simulink model "LF_AC29bus_HVDCdemo_V2_1"  (R2019b)
settings: Solver=FixedStepDiscrete  StartTime=0.0  StopTime=fix(6/Ts)*Ts  FixedStep=Ts  RelTol=1e-3
InitFcn:
  | Ts_avg=150e-6;
  | Ts=50e-6;
  | 
  | %Tc_stab = 1/60/5;
  | %Tc_stab = 2/60;
  | Tc_stab = Ts;
  | 
  | 
  | Ts_avg=150e-6;
  | 
  | Ts=50e-6;
  | 
  | % Rectifier AC side :
  | VLL_nom_R = 735e3; % V
  | Fnom_R = 60;           % Hz
  | 
  | % Inverter AC side :
  | VLL_nom_I = 735e3; % V
  | Fnom_I = 60;           % Hz
  | 
  | % DC :
  | Vdc_nom = 500e3;   % V
  | Idc_nom  = 2000;     % A
undefined symbols (not defined in the file): D1, D11, Delta, test_alpha
libraries: powerlib x223, powerlib_meascontrol x57, simulink x22, sps_avr x7
(part 7 of 10)

== system LF_AC29bus_HVDCdemo_V2_1/North-West Network/Regulators2/Turbine  & Excitation Regulators Mac2 ==
  Pref : Inport
  Vref : Inport  Port=2
  Vm : Inport  Port=3
  w : Inport  Port=4
  Pe : Inport  Port=5
  Add : Sum  Inputs=+-
  Complex to Real-Imag : ComplexToRealImag
  Excitation System : sps_avr/Excitation System  tr=20e-3  reg=[ 300, 0.001 ]  exc=[ 1, 0 ]  tgr=[ 0, 0 ]  damp=[ 0.001, 0.1 ]  sat=[ 0, 0 ]  lim=[ -11.5, 11.5, 0 ]  v0=[1 1.33]
      settings: SourceProductName=Simscape Electrical  SourceProductBaseCode=PS
  Hydraulic Turbine and Governor : powerlib/Machines/Hydraulic Turbine and Governor  sm="[ 10/3  0.07 ]"  gate="[  0.01  0.97518  -0.1  0.1 ]"  reg="[  0.05 1.163  0.105  0  0.01  ]"  hyd="[  0  2.67  ]"  dref=0  po=0.82009
      settings: SourceProductName=Simscape Electrical  SourceProductBaseCode=PS
  Stabilisateur : Subsystem
  Terminator : Terminator
  wref : Constant
  wref1 : Constant
  Pm : Outport
  Vf : Outport  Port=2
  wires:
  Stabilisateur/1(Stab) -> Excitation System/4
  Add/1 -> Stabilisateur/3(dw), Hydraulic Turbine and Governor/5
  wref1/1 -> Add/2
  Complex to Real-Imag/1 -> Excitation System/2
  Complex to Real-Imag/2 -> Excitation System/3
  Vm/1 -> Complex to Real-Imag/1
  w/1 -> Add/1, Hydraulic Turbine and Governor/3
  wref/1 -> Hydraulic Turbine and Governor/1
  Vref/1 -> Excitation System/1
  Pref/1 -> Hydraulic Turbine and Governor/2
  Pe/1 -> Stabilisateur/2(Pe), Hydraulic Turbine and Governor/4
  Excitation System/1 -> Vf/1
  Hydraulic Turbine and Governor/1 -> Stabilisateur/1(Pm), Pm/1
  Hydraulic Turbine and Governor/2 -> Terminator/1

== system LF_AC29bus_HVDCdemo_V2_1/North-West Network/Regulators3/Turbine  & Excitation Regulators Mac2 ==
  Pref : Inport
  Vref : Inport  Port=2
  Vm : Inport  Port=3
  w : Inport  Port=4
  Pe : Inport  Port=5
  Add : Sum  Inputs=+-
  Complex to Real-Imag : ComplexToRealImag
  Excitation System : sps_avr/Excitation System  tr=20e-3  reg=[ 300, 0.001 ]  exc=[ 1, 0 ]  tgr=[ 0, 0 ]  damp=[ 0.001, 0.1 ]  sat=[ 0, 0 ]  lim=[ -11.5, 11.5, 0 ]  v0=[1 1.3999]
      settings: SourceProductName=Simscape Electrical  SourceProductBaseCode=PS
  Hydraulic Turbine and Governor : powerlib/Machines/Hydraulic Turbine and Governor  sm="[ 10/3  0.07 ]"  gate="[  0.01  0.97518  -0.1  0.1 ]"  reg="[  0.05 1.163  0.105  0  0.01  ]"  hyd="[  0  2.67  ]"  dref=0  po=0.90231
      settings: SourceProductName=Simscape Electrical  SourceProductBaseCode=PS
  Stabilisateur : Subsystem
  Terminator : Terminator
  wref : Constant
  wref1 : Constant
  Pm : Outport
  Vf : Outport  Port=2
  wires:
  Hydraulic Turbine and Governor/2 -> Terminator/1
  Hydraulic Turbine and Governor/1 -> Pm/1, Stabilisateur/1(Pm)
  Excitation System/1 -> Vf/1
  Pe/1 -> Hydraulic Turbine and Governor/4, Stabilisateur/2(Pe)
  Pref/1 -> Hydraulic Turbine and Governor/2
  Vref/1 -> Excitation System/1
  wref/1 -> Hydraulic Turbine and Governor/1
  w/1 -> Hydraulic Turbine and Governor/3, Add/1
  Vm/1 -> Complex to Real-Imag/1
  Complex to Real-Imag/2 -> Excitation System/3
  Complex to Real-Imag/1 -> Excitation System/2
  wref1/1 -> Add/2
  Add/1 -> Hydraulic Turbine and Governor/5, Stabilisateur/3(dw)
  Stabilisateur/1(Stab) -> Excitation System/4

== system LF_AC29bus_HVDCdemo_V2_1/North-West Network/Regulators4/Turbine  & Excitation Regulators Mac2 ==
  Pref : Inport
  Vref : Inport  Port=2
  Vm : Inport  Port=3
  w : Inport  Port=4
  Pe : Inport  Port=5
  Add : Sum  Inputs=+-
  Complex to Real-Imag : ComplexToRealImag
  Excitation System : sps_avr/Excitation System  tr=20e-3  reg=[ 300, 0.001 ]  exc=[ 1, 0 ]  tgr=[ 0, 0 ]  damp=[ 0.001, 0.1 ]  sat=[ 0, 0 ]  lim=[ -11.5, 11.5, 0 ]  v0=[1 1.3172]
      settings: SourceProductName=Simscape Electrical  SourceProductBaseCode=PS
  Hydraulic Turbine and Governor : powerlib/Machines/Hydraulic Turbine and Governor  sm="[ 10/3  0.07 ]"  gate="[  0.01  0.97518  -0.1  0.1 ]"  reg="[  0.05 1.163  0.105  0  0.01  ]"  hyd="[  0  2.67  ]"  dref=0  po=0.92839
      settings: SourceProductName=Simscape Electrical  SourceProductBaseCode=PS
  Stabilisateur : Subsystem
  Terminator : Terminator
  wref : Constant
  wref1 : Constant
  Pm : Outport
  Vf : Outport  Port=2
  wires:
  Stabilisateur/1(Stab) -> Excitation System/4
  Add/1 -> Stabilisateur/3(dw), Hydraulic Turbine and Governor/5
  wref1/1 -> Add/2
  Complex to Real-Imag/1 -> Excitation System/2
  Complex to Real-Imag/2 -> Excitation System/3
  Vm/1 -> Complex to Real-Imag/1
  w/1 -> Add/1, Hydraulic Turbine and Governor/3
  wref/1 -> Hydraulic Turbine and Governor/1
  Vref/1 -> Excitation System/1
  Pref/1 -> Hydraulic Turbine and Governor/2
  Pe/1 -> Stabilisateur/2(Pe), Hydraulic Turbine and Governor/4
  Excitation System/1 -> Vf/1
  Hydraulic Turbine and Governor/1 -> Stabilisateur/1(Pm), Pm/1
  Hydraulic Turbine and Governor/2 -> Terminator/1

== system LF_AC29bus_HVDCdemo_V2_1/North_East Network/Regulateurs6/Turbine  & Excitation Regulators Mac2 ==
  Pref : Inport
  Vref : Inport  Port=2
  Vm : Inport  Port=3
  w : Inport  Port=4
  Pe : Inport  Port=5
  Add : Sum  Inputs=+-
  Complex to Real-Imag : ComplexToRealImag
  Excitation System : sps_avr/Excitation System  tr=20e-3  reg=[ 300, 0.001 ]  exc=[ 1, 0 ]  tgr=[ 0, 0 ]  damp=[ 0.001, 0.1 ]  sat=[ 0, 0 ]  lim=[ -11.5, 11.5, 0 ]  v0=[1 1.2956]
      settings: SourceProductName=Simscape Electrical  SourceProductBaseCode=PS
  Hydraulic Turbine and Governor : powerlib/Machines/Hydraulic Turbine and Governor  sm="[ 10/3  0.07 ]"  gate="[  0.01  0.97518  -0.1  0.1 ]"  reg="[  0.05 1.163  0.105  0  0.01  ]"  hyd="[  0  2.67  ]"  dref=0  po=0.89515
      settings: SourceProductName=Simscape Electrical  SourceProductBaseCode=PS
  Stabilisateur : Subsystem
  Terminator : Terminator
  wref : Constant
  wref1 : Constant
  Pm : Outport
  Vf : Outport  Port=2
  wires:
  Hydraulic Turbine and Governor/2 -> Terminator/1
  Hydraulic Turbine and Governor/1 -> Pm/1, Stabilisateur/1(Pm)
  Excitation System/1 -> Vf/1
  Pe/1 -> Hydraulic Turbine and Governor/4, Stabilisateur/2(Pe)
  Pref/1 -> Hydraulic Turbine and Governor/2
  Vref/1 -> Excitation System/1
  wref/1 -> Hydraulic Turbine and Governor/1
  w/1 -> Hydraulic Turbine and Governor/3, Add/1
  Vm/1 -> Complex to Real-Imag/1
  Complex to Real-Imag/2 -> Excitation System/3
  Complex to Real-Imag/1 -> Excitation System/2
  wref1/1 -> Add/2
  Add/1 -> Hydraulic Turbine and Governor/5, Stabilisateur/3(dw)
  Stabilisateur/1(Stab) -> Excitation System/4

== system LF_AC29bus_HVDCdemo_V2_1/North_East Network/Regulateurs7/Turbine  & Excitation Regulators Mac2 ==
  Pref : Inport
  Vref : Inport  Port=2
  Vm : Inport  Port=3
  w : Inport  Port=4
  Pe : Inport  Port=5
  Add : Sum  Inputs=+-
  Complex to Real-Imag : ComplexToRealImag
  Excitation System : sps_avr/Excitation System  tr=20e-3  reg=[ 300, 0.001 ]  exc=[ 1, 0 ]  tgr=[ 0, 0 ]  damp=[ 0.001, 0.1 ]  sat=[ 0, 0 ]  lim=[ -11.5, 11.5, 0 ]  v0=[1 1.1895]
      settings: SourceProductName=Simscape Electrical  SourceProductBaseCode=PS
  Hydraulic Turbine and Governor : powerlib/Machines/Hydraulic Turbine and Governor  sm="[ 10/3  0.07 ]"  gate="[  0.01  0.97518  -0.1  0.1 ]"  reg="[  0.05 1.163  0.105  0  0.01  ]"  hyd="[  0  2.67  ]"  dref=0  po=0.90241
      settings: SourceProductName=Simscape Electrical  SourceProductBaseCode=PS
  Stabilisateur : Subsystem
  Terminator : Terminator
  wref : Constant
  wref1 : Constant
  Pm : Outport
  Vf : Outport  Port=2
  wires:
  Stabilisateur/1(Stab) -> Excitation System/4
  Add/1 -> Stabilisateur/3(dw), Hydraulic Turbine and Governor/5
  wref1/1 -> Add/2
  Complex to Real-Imag/1 -> Excitation System/2
  Complex to Real-Imag/2 -> Excitation System/3
  Vm/1 -> Complex to Real-Imag/1
  w/1 -> Add/1, Hydraulic Turbine and Governor/3
  wref/1 -> Hydraulic Turbine and Governor/1
  Vref/1 -> Excitation System/1
  Pref/1 -> Hydraulic Turbine and Governor/2
  Pe/1 -> Stabilisateur/2(Pe), Hydraulic Turbine and Governor/4
  Excitation System/1 -> Vf/1
  Hydraulic Turbine and Governor/1 -> Stabilisateur/1(Pm), Pm/1
  Hydraulic Turbine and Governor/2 -> Terminator/1

== system LF_AC29bus_HVDCdemo_V2_1/Regulators/Turbine  & Excitation Regulators Mac2/Stabilisateur ==
  Pm : Inport
  Pe : Inport  Port=2
  dw : Inport  Port=3
  Generic Power System Stabilizer : powerlib/Machines/Generic Power System Stabilizer  Tsensor=15e-3  K=2.5  Twashout=1  Tleadlag1="[0.06  1]"  Tleadlag2="[0  0]"  VSlimits=[-0.15 0.15]  Vinit=0  Plot_On=off  MagdB_On=on  FreqRange=logspace(-2,2,500)
      settings: SourceProductName=Simscape Electrical  SourceProductBaseCode=PS
  Ground1 : Ground
  Multi-Band Power System Stabilizer : powerlib/Machines/Multi-Band Power System Stabilizer  OperationMode=Simplified settings  Kg=0.7  GL=[0.2 10]  GI=[0.9 30]  GH=[12.0 115]  GLd=[66 66 9.4]  TcLF=[1.667 2 0 0 0 0 2 2.4 0 0 0 0 1 1]  GId=[66 66 47.6]  TcIF=[1 1 0.25 0.3 0 0 1 1 0.3 0.36 0 0 0 0]  GHd=[66 66 233]  TcHF="[0.01 0.012 0 0 0 0  0.012 0.0144 0 0 0 0 1 1]"  LIM=[.075 .15 .15 .15]  Plot_On=off  MagdB_On=on  FreqRange=logspace(-2,2,500)
      settings: SourceProductName=Simscape Electrical  SourceProductBaseCode=PS
  Multiport Switch : MultiPortSwitch  SaturateOnIntegerOverflow=on  InputSameDT=on
  Sum2 : Sum  Inputs=+-  SaturateOnIntegerOverflow=on  InputSameDT=on  OutDataTypeStr=Inherit: Same as first input
  Stab : Outport  InitialOutput=0
  wires:
  Multi-Band Power System Stabilizer/1 -> Multiport Switch/4
  dw/1 -> Multi-Band Power System Stabilizer/1
  [PSS_select] -> Multiport Switch/1
  Ground1/1 -> Multiport Switch/2
  Pe/1 -> Sum2/2
  Pm/1 -> Sum2/1
  Sum2/1 -> Generic Power System Stabilizer/1
  Generic Power System Stabilizer/1 -> Multiport Switch/3
  Multiport Switch/1 -> Stab/1

== system LF_AC29bus_HVDCdemo_V2_1/HVDC_network_avg/Inverter Average model/HVDC_CONV_AVG/3-phase Current Source ==
  note: Ic = -(Ia + Ib)
  Iab : Inport
  Controlled Current Source : powerlib/Electrical Sources/Controlled Current Source  Initialize=off  Source_Type=AC  Amplitude=0  Phase=0  Frequency=0  Measurements=None
      settings: SourceProductName=Simscape Electrical
  Controlled Current Source1 : powerlib/Electrical Sources/Controlled Current Source  Initialize=off  Source_Type=AC  Amplitude=0  Phase=0  Frequency=0  Measurements=None
      settings: SourceProductName=Simscape Electrical
  Demux : Demux  Outputs=2
  A : PMIOPort  Side=Left
  B : PMIOPort  Port=2  Side=Left
  C : PMIOPort  Port=3  Side=Left
  wires:
  Iab/1 -> Demux/1
  Demux/1 -> Controlled Current Source/1
  Demux/2 -> Controlled Current Source1/1
  connections:
  A/RConn1 -- Controlled Current Source/LConn1
  B/RConn1 -- Controlled Current Source1/LConn1
  C/RConn1 -- Controlled Current Source1/RConn1 -- Controlled Current Source/RConn1

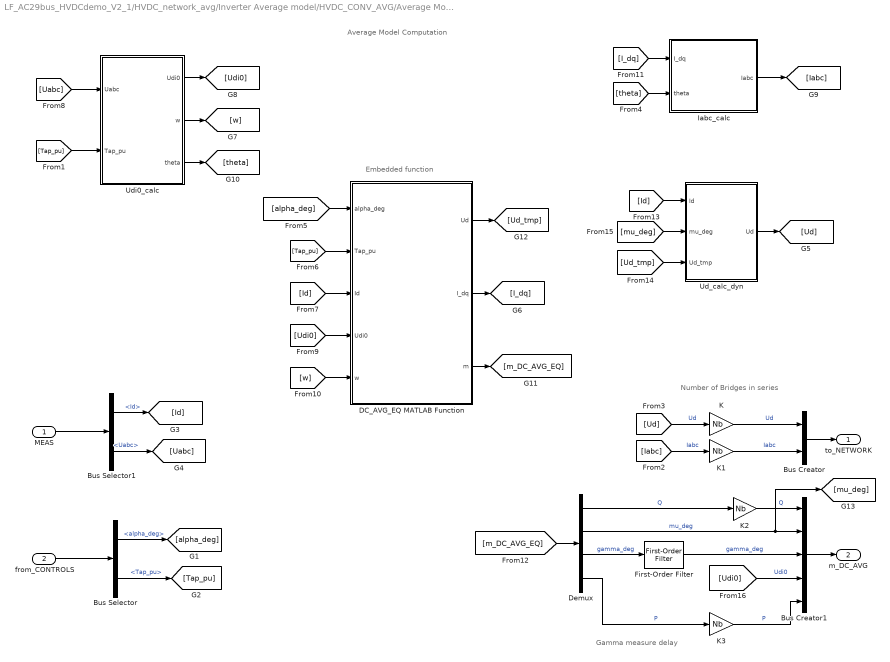
== system LF_AC29bus_HVDCdemo_V2_1/HVDC_network_avg/Inverter Average model/HVDC_CONV_AVG/Average Model Computation ==
  note: Embedded function
  note: Gamma measure delay
  note: Average Model Computation
  note: Number of Bridges
      | in series
  MEAS : Inport
  from_CONTROLS : Inport  Port=2
  Bus Creator : BusCreator  Inputs=2
  Bus Creator1 : BusCreator  Inputs=5
  Bus Selector : BusSelector  OutputSignals=alpha_deg,Tap_pu
  Bus Selector1 : BusSelector  OutputSignals=Id,Uabc
  DC_AVG_EQ MATLAB Function : MATLAB Function  TreatAsAtomicUnit=on
  Demux : Demux
  First-Order Filter : powerlib_meascontrol/Filters/First-Order Filter  FilterType=Lowpass  Tc=1/(6*fn*2*pi)  Ts=Ts  Initialize=off  Vac_Init=[0, 0, 60]  Vdc_Init=0  PlotResponse=off  FreqRange="[0,  200,  1]"
      settings: SourceProductName=Simscape Electrical
  Iabc_calc : Subsystem
  K{,1..3} (4 alike) : Gain  Gain=Nb
  Ud_calc_dyn : Subsystem
  Udi0_calc : Subsystem
  to_NETWORK : Outport
  m_DC_AVG : Outport  Port=2
  wires:
  K3/1 -> Bus Creator1/5  "P"
  Demux/4 -> K3/1  "P"
  First-Order Filter/1 -> Bus Creator1/3  "gamma_deg"
  Demux/3 -> First-Order Filter/1  "gamma_deg"
  [Udi0] -> Bus Creator1/4  "Udi0"
  [mu_deg] -> Ud_calc_dyn/2(mu_deg)
  [Ud_tmp] -> Ud_calc_dyn/3(Ud_tmp)
  DC_AVG_EQ MATLAB Function/1(Ud) -> [Ud_tmp]
  Ud_calc_dyn/1(Ud) -> [Ud]
  [Id] -> Ud_calc_dyn/1(Id)
  K2/1 -> Bus Creator1/1  "Q"
  [w] -> DC_AVG_EQ MATLAB Function/5(w)
  [Udi0] -> DC_AVG_EQ MATLAB Function/4(Udi0)
  [Id] -> DC_AVG_EQ MATLAB Function/3(Id)
  [Uabc] -> Udi0_calc/1(Uabc)
  Bus Selector/1 -> [alpha_deg]  "<alpha_deg>"
  from_CONTROLS/1 -> Bus Selector/1
  Bus Selector/2 -> [Tap_pu]  "<Tap_pu>"
  MEAS/1 -> Bus Selector1/1
  Bus Selector1/1 -> [Id]  "<Id>"
  Bus Selector1/2 -> [Uabc]  "<Uabc>"
  [Tap_pu] -> Udi0_calc/2(Tap_pu)
  Bus Creator/1 -> to_NETWORK/1
  [Iabc] -> K1/1  "Iabc"
  [Ud] -> K/1  "Ud"
  K/1 -> Bus Creator/1  "Ud"
  K1/1 -> Bus Creator/2  "Iabc"
  Udi0_calc/2(w) -> [w]
  Udi0_calc/1(Udi0) -> [Udi0]
  Iabc_calc/1(Iabc) -> [Iabc]
  Udi0_calc/3(theta) -> [theta]
  [theta] -> Iabc_calc/2(theta)
  [I_dq] -> Iabc_calc/1(I_dq)
  [alpha_deg] -> DC_AVG_EQ MATLAB Function/1(alpha_deg)
  [Tap_pu] -> DC_AVG_EQ MATLAB Function/2(Tap_pu)
  DC_AVG_EQ MATLAB Function/2(I_dq) -> [I_dq]
  DC_AVG_EQ MATLAB Function/3(m) -> [m_DC_AVG_EQ]
  [m_DC_AVG_EQ] -> Demux/1
  Demux/1 -> K2/1  "Q"
  Demux/2 -> [mu_deg], Bus Creator1/2  "mu_deg"
  Bus Creator1/1 -> m_DC_AVG/1

== system LF_AC29bus_HVDCdemo_V2_1/HVDC_network_avg/Inverter Average model/HVDC_CONV_AVG/CF_alarm ==
  note: CF_alarm
  note: Converter is deblocked
  Pd : Inport
  Udi0 : Inport  Port=2
  gamma_deg : Inport  Port=3
  Abs : Abs
  KPn : Constant  Value=Pn*Nb*0.05
  Logical Operator : Logic  Operator=OR  AllPortsSameDT=off  OutDataTypeStr=boolean
  Logical Operator1 : Logic  AllPortsSameDT=off  OutDataTypeStr=boolean
  Monostable : powerlib_meascontrol/Logic/Monostable  EdgeDetect=Rising  PulseDuration=T_alarm  ic=0  Ts=Ts
      settings: SourceProductName=Simscape Electrical  SourceProductBaseCode=PS
  Off Delay1 (T=1.2/(2*fn)) : powerlib_meascontrol/Logic/On Delay  DelayType=Off delay  delay=1.2/(2*fn)  ic=0  Ts=Ts
      settings: SourceProductName=Simscape Electrical
  Off Delay2 : powerlib_meascontrol/Logic/On Delay  DelayType=Off delay  delay=0.1  ic=0  Ts=Ts
      settings: SourceProductName=Simscape Electrical
  On Delay1 (T=2*Ts) : powerlib_meascontrol/Logic/On Delay  DelayType=On delay  delay=2*Ts  ic=0  Ts=Ts
      settings: SourceProductName=Simscape Electrical
  On Delay2 (T=1.5/(2*fn)) : powerlib_meascontrol/Logic/On Delay  DelayType=On delay  delay=1.5/(2*fn)  ic=0  Ts=Ts
      settings: SourceProductName=Simscape Electrical
  On Delay3 (T=1/fn) : powerlib_meascontrol/Logic/On Delay  DelayType=On delay  delay=1/fn  ic=0  Ts=Ts
      settings: SourceProductName=Simscape Electrical
  Relational Operator : RelationalOperator  Operator=<=  OutDataTypeStr=boolean  RndMeth=Nearest
  Relational Operator1 : RelationalOperator  Operator=<=  OutDataTypeStr=boolean  RndMeth=Nearest
  Relational Operator2 : RelationalOperator  OutDataTypeStr=boolean  RndMeth=Nearest
  Uac_min_lim : Constant  Value=0.8
  Udio_V->pu : Gain  Gain=1/((3*sqrt(2)/pi) * Usec)
  gamma_min_lim : Constant  Value=10
  CF_alarm : Outport
  wires:
  Off Delay2/1 -> Logical Operator1/2
  Abs/1 -> Relational Operator2/1
  Logical Operator1/1 -> Logical Operator/1
  On Delay2 (T=1.5/(2*fn))/1 -> Logical Operator1/1  "low_ac"
  Relational Operator2/1 -> Off Delay2/1
  KPn/1 -> Relational Operator2/2
  Pd/1 -> Abs/1
  On Delay3 (T=1/fn)/1 -> Logical Operator/2  "gamm_lim"
  Relational Operator1/1 -> On Delay3 (T=1/fn)/1
  gamma_min_lim/1 -> Relational Operator1/2
  gamma_deg/1 -> Relational Operator1/1
  Udio_V->pu/1 -> Relational Operator/1
  Uac_min_lim/1 -> Relational Operator/2
  Udi0/1 -> Udio_V->pu/1
  Relational Operator/1 -> On Delay1 (T=2*Ts)/1
  Off Delay1 (T=1.2/(2*fn))/1 -> On Delay2 (T=1.5/(2*fn))/1
  On Delay1 (T=2*Ts)/1 -> Off Delay1 (T=1.2/(2*fn))/1
  Logical Operator/1 -> Monostable/1
  Monostable/1 -> CF_alarm/1

== system LF_AC29bus_HVDCdemo_V2_1/HVDC_network_avg/Inverter Control and Protection (Average model)/Inverter Pole Control (Current//Voltage//Gamma)/Alpha Control ==
  note: Alpha Control
  Forced_alpha : Inport
  D_alpha : Inport  Port=2
  Constant1 : Constant  Value=alpha_min
  Constant2 : Constant  Value=alpha_max
  Constant3 : Constant  Value=test_alpha
  Data Type Conversion : DataTypeConversion  OutDataTypeStr=boolean  SaturateOnIntegerOverflow=on  RndMeth=Zero
  Logical Operator : Logic  Operator=OR
  "Rate Limiter (Rate limit) " : RateLimiter  RisingSlewLimit=PRate_fix  FallingSlewLimit=NRate_fix
  "Rate Limiter (Rate limit)    " : RateLimiter  RisingSlewLimit=PRate_fix  FallingSlewLimit=NRate_fix
  Sum : Sum  Inputs=-+  SaturateOnIntegerOverflow=on  InputSameDT=on  OutDataTypeStr=Inherit: Same as first input
  Switch : Switch  Criteria=u2 > Threshold  SaturateOnIntegerOverflow=on  InputSameDT=on
  Switch1 : Switch  Criteria=u2 > Threshold  SaturateOnIntegerOverflow=on  InputSameDT=on
  fixed alpha (deg) : Constant  Value=alpha_fix
  Max_i : Outport
  Min_i : Outport  Port=2
  wires:
  "Rate Limiter (Rate limit)    "/1 -> Min_i/1
  "Rate Limiter (Rate limit) "/1 -> Max_i/1
  D_alpha/1 -> Sum/1
  Sum/1 -> Switch/3
  Constant2/1 -> Sum/2
  Constant3/1 -> Logical Operator/1
  Logical Operator/1 -> Switch/2, Switch1/2
  Constant1/1 -> Switch1/3
  Switch/1 -> "Rate Limiter (Rate limit) "/1
  Switch1/1 -> "Rate Limiter (Rate limit)    "/1
  fixed alpha (deg)/1 -> Switch/1, Switch1/1
  Forced_alpha/1 -> Data Type Conversion/1
  Data Type Conversion/1 -> Logical Operator/2

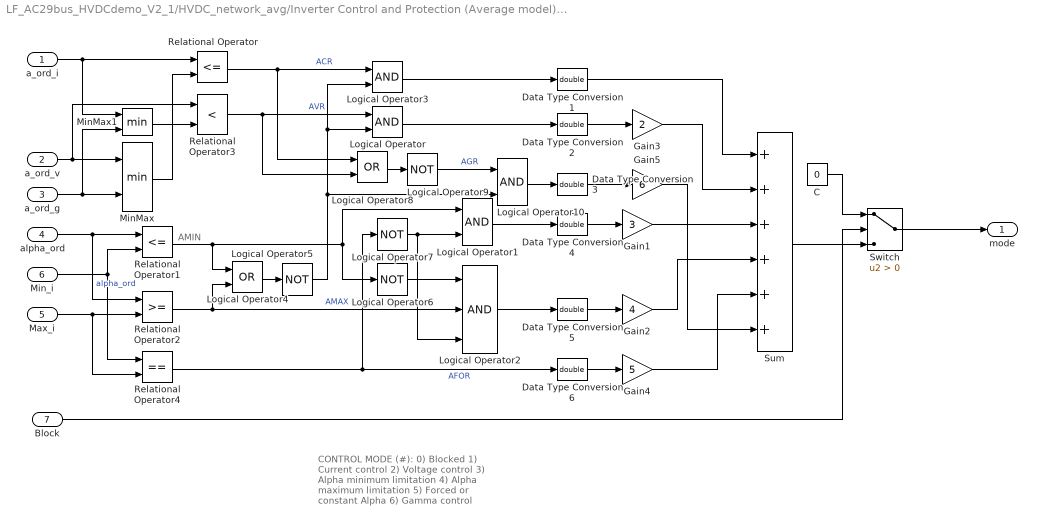
== system LF_AC29bus_HVDCdemo_V2_1/HVDC_network_avg/Inverter Control and Protection (Average model)/Inverter Pole Control (Current//Voltage//Gamma)/Control Mode  ==
  note: AMIN
  note: CONTROL MODE (#):
      |
      | 0) Blocked
      | 1) Current control
      | 2) Voltage control
      | 3) Alpha minimum limitation
      | 4) Alpha maximum limitation
      | 5) Forced or constant Alpha
      | 6) Gamma control
  "a_ord_i " : Inport
  a_ord_v : Inport  Port=2
  a_ord_g : Inport  Port=3
  alpha_ord : Inport  Port=4
  Max_i : Inport  Port=5
  Min_i : Inport  Port=6
  Block : Inport  Port=7
  C : Constant  Value=0
  Data Type Conversion{1..6} (6 alike) : DataTypeConversion  OutDataTypeStr=double
  Gain1 : Gain  Gain=3  OutDataTypeStr=double  SaturateOnIntegerOverflow=on  ParamDataTypeStr=Inherit: Same as input
  Gain2 : Gain  Gain=4  OutDataTypeStr=double  SaturateOnIntegerOverflow=on  ParamDataTypeStr=Inherit: Same as input
  Gain3 : Gain  Gain=2  OutDataTypeStr=double  SaturateOnIntegerOverflow=on  ParamDataTypeStr=Inherit: Same as input
  Gain4 : Gain  Gain=5  OutDataTypeStr=double  SaturateOnIntegerOverflow=on  ParamDataTypeStr=Inherit: Same as input
  Gain5 : Gain  Gain=6  OutDataTypeStr=double  SaturateOnIntegerOverflow=on  ParamDataTypeStr=Inherit: Same as input
  Logical Operator{,1,3,10} (4 alike) : Logic
  Logical Operator2 : Logic  Inputs=3
  Logical Operator4 : Logic  Operator=OR
  Logical Operator{5..7,9} (4 alike) : Logic  Operator=NOT
  Logical Operator8 : Logic  Operator=OR
  MinMax : MinMax  Inputs=2  SaturateOnIntegerOverflow=on  InputSameDT=on
  MinMax1 : MinMax  Inputs=2  SaturateOnIntegerOverflow=on  InputSameDT=on
  Relational Operator : RelationalOperator  Operator=<=  RndMeth=Nearest  InputSameDT=on
  Relational Operator1 : RelationalOperator  Operator=<=  RndMeth=Nearest  InputSameDT=on
  Relational Operator2 : RelationalOperator  RndMeth=Nearest  InputSameDT=on
  Relational Operator3 : RelationalOperator  Operator=<  RndMeth=Nearest  InputSameDT=on
  Relational Operator4 : RelationalOperator  Operator===  RndMeth=Nearest  InputSameDT=on
  Sum : Sum  Inputs=++++++  SaturateOnIntegerOverflow=on  InputSameDT=on  OutDataTypeStr=Inherit: Same as first input
  Switch : Switch  Criteria=u2 > Threshold  SaturateOnIntegerOverflow=on  InputSameDT=on
  mode : Outport
  wires:
  Data Type Conversion6/1 -> Gain4/1
  Data Type Conversion5/1 -> Gain2/1
  Data Type Conversion4/1 -> Gain1/1
  Data Type Conversion3/1 -> Gain5/1
  Data Type Conversion2/1 -> Gain3/1
  Data Type Conversion1/1 -> Sum/1
  Switch/1 -> mode/1
  Logical Operator5/1 -> Logical Operator3/2, Logical Operator/2, Logical Operator10/2
  Logical Operator7/1 -> Logical Operator2/3, Logical Operator1/2
  Gain4/1 -> Sum/5
  Logical Operator1/1 -> Data Type Conversion4/1
  Relational Operator4/1 -> Logical Operator7/1, Data Type Conversion6/1  "AFOR"
  Max_i/1 -> Relational Operator4/2, Relational Operator2/2
  Min_i/1 -> Relational Operator4/1, Relational Operator1/2
  Gain2/1 -> Sum/4
  Gain1/1 -> Sum/3
  Logical Operator2/1 -> Data Type Conversion5/1
  Logical Operator6/1 -> Logical Operator2/1
  Relational Operator2/1 -> Logical Operator2/2, Logical Operator4/2  "AMAX"
  Logical Operator4/1 -> Logical Operator5/1
  Relational Operator1/1 -> Logical Operator1/1, Logical Operator6/1, Logical Operator4/1
  alpha_ord/1 -> Relational Operator2/1, Relational Operator1/1  "alpha_ord"
  Logical Operator/1 -> Data Type Conversion2/1
  Relational Operator3/1 -> Logical Operator/1, Logical Operator8/2  "AVR"
  Gain3/1 -> Sum/2
  Logical Operator3/1 -> Data Type Conversion1/1
  Relational Operator/1 -> Logical Operator3/1, Logical Operator8/1  "ACR"
  "a_ord_i "/1 -> Relational Operator/1, MinMax1/1
  Block/1 -> Switch/2
  Sum/1 -> Switch/3
  C/1 -> Switch/1
  a_ord_v/1 -> MinMax/1, Relational Operator3/1
  a_ord_g/1 -> MinMax/2, MinMax1/2
  MinMax/1 -> Relational Operator/2
  Logical Operator8/1 -> Logical Operator9/1
  Gain5/1 -> Sum/6
  MinMax1/1 -> Relational Operator3/2
  Logical Operator9/1 -> Logical Operator10/1  "AGR"
  Logical Operator10/1 -> Data Type Conversion3/1

== system LF_AC29bus_HVDCdemo_V2_1/HVDC_network_avg/Inverter Control and Protection (Average model)/Inverter Pole Control (Current//Voltage//Gamma)/Current Regulator ==
  note: Current Regulator
  Max_i : Inport
  Min_i : Inport  Port=2
  ERR : Inport  Port=3
  Max_pi : Inport  Port=4
  Min_pi : Inport  Port=5
  Alpha_lin : Inport  Port=6
  Max_lin : Inport  Port=7
  Min_lin : Inport  Port=8
  Inv : Inport  Port=9
  PI Regulator with external limits and linrarized Kp (Discrete) : Subsystem  mask(PI Regulator  With  External  Limits (Discrete)){Kp=Kp_I, Ki=Ki_I, IC_i=ICi_I, On_lin=on, pas=Ts}
      mask prompts: Kp "Kp (deg/pu):"; Ki "Ki (deg/pu/s):"; IC_i "Integrator Initial Condition (deg):"; On_lin "Linearization  (On)"; pas "Sample time (s):"
      mask help: For the linearization it is important to specifie the mode of operation i.e. rectifier or inverter (negation of rectifier).
      mask Display: disp('PI Regulator\nWith external limits\n(Linearized Kp)\n(Discrete)\n\n')
  Alpha_ord : Outport
  wires:
  PI Regulator with external limits and linrarized Kp (Discrete)/1(Alpha_ord) -> Alpha_ord/1
  Max_i/1 -> PI Regulator with external limits and linrarized Kp (Discrete)/1(Max_i)
  Min_i/1 -> PI Regulator with external limits and linrarized Kp (Discrete)/2(Min_i)
  ERR/1 -> PI Regulator with external limits and linrarized Kp (Discrete)/3(ERR)
  Max_pi/1 -> PI Regulator with external limits and linrarized Kp (Discrete)/4(Max_pi)
  Min_pi/1 -> PI Regulator with external limits and linrarized Kp (Discrete)/5(Min_pi)
  Alpha_lin/1 -> PI Regulator with external limits and linrarized Kp (Discrete)/6(Alpha_lin)
  Max_lin/1 -> PI Regulator with external limits and linrarized Kp (Discrete)/7(Max_lin)
  Min_lin/1 -> PI Regulator with external limits and linrarized Kp (Discrete)/8(Min_lin)
  Inv/1 -> PI Regulator with external limits and linrarized Kp (Discrete)/9(Inv)

== system LF_AC29bus_HVDCdemo_V2_1/HVDC_network_avg/Inverter Control and Protection (Average model)/Inverter Pole Control (Current//Voltage//Gamma)/Gamma Error ==
  note: Gamma Error
  G_ref : Inport
  G_meas : Inport  Port=2
  Block : Inport  Port=3
  Id_err : Inport  Port=4
  Enable (Held) : EnablePort  PropagateVarSize=During execution
  Constant1 : Constant  Value=0
  Constant2 : Constant  Value=0
  Constant3 : Constant  Value=G_marg
  Constant4 : Constant  Value=Id_marg
  First-Order Filter (T=0.01) : powerlib_meascontrol/Filters/First-Order Filter  FilterType=Lowpass  Tc=0.01  Ts=Ts  Initialize=off  Vac_Init=[0, 0, 60]  Vdc_Init=0  PlotResponse=off  FreqRange="[0,  200,  1]"
      settings: SourceProductName=Simscape Electrical
  MIN:eps MAX:inf : Saturate  UpperLimit=inf  LowerLimit=eps
  Math Function : Math  Operator=reciprocal  SaturateOnIntegerOverflow=on
  Product1 : Product  Inputs=3  SaturateOnIntegerOverflow=on  InputSameDT=on  OutDataTypeStr=Inherit: Same as first input
  Saturation Dynamic : simulink/Discontinuities/Saturation Dynamic  OutMin=[]  OutMax=[]  OutDataTypeStr=Inherit: Same as second input  OutDataType=fixdt(1, 16)  OutScaling=2^-10  DoSatur=off
  Sum3 : Sum  Inputs=-+-  SaturateOnIntegerOverflow=on  InputSameDT=on  OutDataTypeStr=Inherit: Same as first input
  Switch2 : Switch  Criteria=u2 > Threshold  SaturateOnIntegerOverflow=on  InputSameDT=on
  ERR_G : Outport
  wires:
  Saturation Dynamic/1 -> Product1/3
  Sum3/1 -> Switch2/3
  G_ref/1 -> Sum3/1
  G_meas/1 -> Sum3/2
  Constant1/1 -> Switch2/1
  Block/1 -> Switch2/2
  Switch2/1 -> ERR_G/1  "ERR"
  Constant2/1 -> Saturation Dynamic/3
  Math Function/1 -> Product1/2
  MIN:eps MAX:inf/1 -> Math Function/1
  Constant4/1 -> MIN:eps MAX:inf/1, Saturation Dynamic/1
  Product1/1 -> First-Order Filter (T=0.01)/1
  First-Order Filter (T=0.01)/1 -> Sum3/3  "dG"
  Id_err/1 -> Saturation Dynamic/2
  Constant3/1 -> Product1/1

== system LF_AC29bus_HVDCdemo_V2_1/HVDC_network_avg/Inverter Control and Protection (Average model)/Inverter Pole Control (Current//Voltage//Gamma)/Gamma Regulator ==
  note: Gamma Regulator
  Max_i : Inport
  Min_i : Inport  Port=2
  ERR : Inport  Port=3
  Max_pi : Inport  Port=4
  Min_pi : Inport  Port=5
  Alpha_lin : Inport  Port=6
  Max_lin : Inport  Port=7
  Min_lin : Inport  Port=8
  Inv : Inport  Port=9
  Enable (Held) : EnablePort  PropagateVarSize=During execution
  PI Regulator with external limits and linrarized Kp (Discrete)1 : Subsystem  mask(PI Regulator  With  External  Limits (Discrete)){Kp=Kp_G, Ki=Ki_G, IC_i=ICi_G, On_lin=on, pas=Ts}
      mask prompts: Kp "Kp (deg/pu):"; Ki "Ki (deg/pu/s):"; IC_i "Integrator Initial Condition (deg):"; On_lin "Linearization  (On)"; pas "Sample time (s):"
      mask help: For the linearization it is important to specifie the mode of operation i.e. rectifier or inverter (negation of rectifier).
      mask Display: disp('PI Regulator\nWith external limits\n(Linearized Kp)\n(Discrete)\n\n')
  Alpha_ord : Outport
  wires:
  PI Regulator with external limits and linrarized Kp (Discrete)1/1(Alpha_ord) -> Alpha_ord/1
  Max_i/1 -> PI Regulator with external limits and linrarized Kp (Discrete)1/1(Max_i)
  Min_i/1 -> PI Regulator with external limits and linrarized Kp (Discrete)1/2(Min_i)
  ERR/1 -> PI Regulator with external limits and linrarized Kp (Discrete)1/3(ERR)
  Max_pi/1 -> PI Regulator with external limits and linrarized Kp (Discrete)1/4(Max_pi)
  Min_pi/1 -> PI Regulator with external limits and linrarized Kp (Discrete)1/5(Min_pi)
  Alpha_lin/1 -> PI Regulator with external limits and linrarized Kp (Discrete)1/6(Alpha_lin)
  Max_lin/1 -> PI Regulator with external limits and linrarized Kp (Discrete)1/7(Max_lin)
  Min_lin/1 -> PI Regulator with external limits and linrarized Kp (Discrete)1/8(Min_lin)
  Inv/1 -> PI Regulator with external limits and linrarized Kp (Discrete)1/9(Inv)

== system LF_AC29bus_HVDCdemo_V2_1/HVDC_network_avg/Inverter Control and Protection (Average model)/Inverter Pole Control (Current//Voltage//Gamma)/Voltage Error ==
  note: Voltage Error
  Vd_ref : Inport
  Vd_meas : Inport  Port=2
  Block : Inport  Port=3
  Id_err : Inport  Port=4
  Enable (Held) : EnablePort  PropagateVarSize=During execution
  Constant1 : Constant  Value=0
  Constant2 : Constant  Value=0
  Constant3 : Constant  Value=Vd_marg
  Constant4 : Constant  Value=Id_marg
  First-Order Filter (T = 0.1) : powerlib_meascontrol/Filters/First-Order Filter  FilterType=Lowpass  Tc=0.01  Ts=Ts  Initialize=on  Vac_Init=[0, 0, 60]  Vdc_Init=0  PlotResponse=off  FreqRange="[0,  200,  1]"
      settings: SourceProductName=Simscape Electrical
  MIN:eps MAX:inf : Saturate  UpperLimit=inf  LowerLimit=eps
  Math Function : Math  Operator=reciprocal  SaturateOnIntegerOverflow=on
  Product1 : Product  Inputs=3  SaturateOnIntegerOverflow=on  InputSameDT=on  OutDataTypeStr=Inherit: Same as first input
  Saturation Dynamic : simulink/Discontinuities/Saturation Dynamic  OutMin=[]  OutMax=[]  OutDataTypeStr=Inherit: Same as second input  OutDataType=fixdt(1, 16)  OutScaling=2^-10  DoSatur=off
  Sum3 : Sum  Inputs=+--  SaturateOnIntegerOverflow=on  InputSameDT=on  OutDataTypeStr=Inherit: Same as first input
  Switch2 : Switch  Criteria=u2 > Threshold  SaturateOnIntegerOverflow=on  InputSameDT=on
  ERR_V : Outport
  wires:
  Saturation Dynamic/1 -> Product1/3
  Constant3/1 -> Product1/1
  Id_err/1 -> Saturation Dynamic/2
  First-Order Filter (T = 0.1)/1 -> Sum3/3  "dV"
  Product1/1 -> First-Order Filter (T = 0.1)/1
  Constant4/1 -> MIN:eps MAX:inf/1, Saturation Dynamic/1
  MIN:eps MAX:inf/1 -> Math Function/1
  Math Function/1 -> Product1/2
  Constant2/1 -> Saturation Dynamic/3
  Switch2/1 -> ERR_V/1  "ERR"
  Block/1 -> Switch2/2
  Constant1/1 -> Switch2/1
  Vd_meas/1 -> Sum3/2
  Vd_ref/1 -> Sum3/1
  Sum3/1 -> Switch2/3

== system LF_AC29bus_HVDCdemo_V2_1/HVDC_network_avg/Inverter Control and Protection (Average model)/Inverter Pole Control (Current//Voltage//Gamma)/Voltage Regulator ==
  note: Voltage Regulator
  Max_i : Inport
  Min_i : Inport  Port=2
  ERR : Inport  Port=3
  Max_pi : Inport  Port=4
  Min_pi : Inport  Port=5
  Alpha_lin : Inport  Port=6
  Max_lin : Inport  Port=7
  Min_lin : Inport  Port=8
  Inv : Inport  Port=9
  Enable (Held) : EnablePort  PropagateVarSize=During execution
  PI Regulator with external limits and linrarized Kp (Discrete) : Subsystem  mask(PI Regulator  With  External  Limits (Discrete)){Kp=Kp_V, Ki=Ki_V, IC_i=ICi_V, On_lin=on, pas=Ts}
      mask prompts: Kp "Kp (deg/pu):"; Ki "Ki (deg/pu/s):"; IC_i "Integrator Initial Condition (deg):"; On_lin "Linearization  (On)"; pas "Sample time (s):"
      mask help: For the linearization it is important to specifie the mode of operation i.e. rectifier or inverter (negation of rectifier).
      mask Display: disp('PI Regulator\nWith external limits\n(Linearized Kp)\n(Discrete)\n\n')
  Alpha_ord : Outport
  wires:
  Inv/1 -> PI Regulator with external limits and linrarized Kp (Discrete)/9(Inv)
  Min_lin/1 -> PI Regulator with external limits and linrarized Kp (Discrete)/8(Min_lin)
  Max_lin/1 -> PI Regulator with external limits and linrarized Kp (Discrete)/7(Max_lin)
  Alpha_lin/1 -> PI Regulator with external limits and linrarized Kp (Discrete)/6(Alpha_lin)
  Min_pi/1 -> PI Regulator with external limits and linrarized Kp (Discrete)/5(Min_pi)
  Max_pi/1 -> PI Regulator with external limits and linrarized Kp (Discrete)/4(Max_pi)
  ERR/1 -> PI Regulator with external limits and linrarized Kp (Discrete)/3(ERR)
  Min_i/1 -> PI Regulator with external limits and linrarized Kp (Discrete)/2(Min_i)
  Max_i/1 -> PI Regulator with external limits and linrarized Kp (Discrete)/1(Max_i)
  PI Regulator with external limits and linrarized Kp (Discrete)/1(Alpha_ord) -> Alpha_ord/1

== system LF_AC29bus_HVDCdemo_V2_1/HVDC_network_avg/Inverter Control and Protection (Average model)/Inverter Pole Control (Current//Voltage//Gamma)/Voltage dependent Current Order Limiter ==
  note: Voltage dependent Current Order Limiter (VDCOL) (Discrete)
  Id_ref (pu) : Inport
  Vd (pu) : Inport  Port=2
  Constant : Constant  Value=Id_min
  Constant1 : Constant  Value=Vd_min
  Constant2 : Constant  Value=Vd_seuil
  Constant3 : Constant
  Constant4 : Constant
  Constant5 : Constant  Value=Tu
  Logical Operator : Logic  Operator=NOT
  Low Pass (IC = 1.0) : Subsystem  mask(Low Pass Filter With Reset (discrete: Zoh method, Forward Euler)){ic=1, dt=Ts}
      mask prompts: ic "Initial condition:"; dt "Sample time (s)"
      mask help:
      | The output will be reset to the input value (Time constant = 0)  during the input (2) is True. The Time constant (T) is defined by
      | input (3).
      mask Display:
      | plot(0,0,100,100,[90,80,70,60,50,40,29,20,10],[60,55,52,55,60,65,67,65,60],[89,80,71,60,50,40,30,20,10],[40,35,32,35,40,45,47,45,40],[56,44],[70,50]);
      | disp('\n\nD')
  Math Function : Math  Operator=reciprocal  SaturateOnIntegerOverflow=on
  Max = 10 Min=Id_min_abs : Saturate  UpperLimit=10  LowerLimit=Id_min_abs
  MinMax2 : MinMax  Function=max  Inputs=2  SaturateOnIntegerOverflow=on  InputSameDT=on
  MinMax3 : MinMax  Inputs=2  SaturateOnIntegerOverflow=on  InputSameDT=on
  Product{,1..4} (5 alike) : Product  SaturateOnIntegerOverflow=on  InputSameDT=on  OutDataTypeStr=Inherit: Same as first input
  Relational Operator : RelationalOperator  RndMeth=Nearest  InputSameDT=on
  Sum : Sum  Inputs=+-  SaturateOnIntegerOverflow=on  InputSameDT=on  OutDataTypeStr=Inherit: Same as first input
  Sum1 : Sum  Inputs=+-  SaturateOnIntegerOverflow=on  InputSameDT=on  OutDataTypeStr=Inherit: Same as first input
  Sum2 : Sum  Inputs=+-  SaturateOnIntegerOverflow=on  InputSameDT=on  OutDataTypeStr=Inherit: Same as first input
  Sum3 : Sum  SaturateOnIntegerOverflow=on  InputSameDT=on  OutDataTypeStr=Inherit: Same as first input
  Unit Delay : UnitDelay  SampleTime=Ts  HasFrameUpgradeWarning=on
  Id_ref_lim : Outport  InitialOutput=0
  Vd_filt : Outport  Port=2  InitialOutput=0
  wires:
  Relational Operator/1 -> Unit Delay/1
  Max = 10 Min=Id_min_abs/1 -> MinMax2/2
  MinMax2/1 -> MinMax3/2
  Product1/1 -> MinMax2/1  "Idref_lim"
  Constant2/1 -> Product3/1, Sum1/1
  Product/1 -> Product3/2, Product2/1  "A"
  Product3/1 -> Sum2/2
  MinMax3/1 -> Id_ref_lim/1
  Id_ref (pu)/1 -> Product4/2, MinMax3/1, Product1/1
  Product4/1 -> Max = 10 Min=Id_min_abs/1  "min"
  Constant/1 -> Product4/1, Sum/2
  Sum3/1 -> Product1/2
  Product2/1 -> Sum3/2
  Sum2/1 -> Sum3/1  "B"
  Constant4/1 -> Sum2/1
  Math Function/1 -> Product/2
  Sum/1 -> Product/1
  Sum1/1 -> Math Function/1
  Constant1/1 -> Sum1/2
  Constant3/1 -> Sum/1
  Constant5/1 -> Low Pass (IC = 1.0)/3(T)
  Low Pass (IC = 1.0)/1(Out) -> Vd_filt/1, Relational Operator/2, Product2/2
  Vd (pu)/1 -> Relational Operator/1, Low Pass (IC = 1.0)/1(In)
  Unit Delay/1 -> Logical Operator/1
  Logical Operator/1 -> Low Pass (IC = 1.0)/2(R)

== system LF_AC29bus_HVDCdemo_V2_1/HVDC_network_avg/Inverter Control and Protection (Average model)/Inverter Pole Control (Current//Voltage//Gamma)/alpha_init ==
  In1 : Inport  PortDimensions=1
  IC : InitialCondition  Value=min([ICi_V,ICi_I,ICi_G])
  Out1 : Outport
  wires:
  IC/1 -> Out1/1
  In1/1 -> IC/1

== system LF_AC29bus_HVDCdemo_V2_1/HVDC_network_avg/Inverter Control and Protection (Average model)/Inverter Protections/Commutation Failure Prevention Control (CFPREV) ==
  note: Commutation failure Prevention Control Module (CFPREV)
  Uabc (pu) : Inport
  C : Constant  Value=STATE
  CFPREV : Subsystem  TreatAsAtomicUnit=on
  AMIN_CFPREV (deg) : Outport
  wires:
  C/1 -> CFPREV/Enable
  Uabc (pu)/1 -> CFPREV/1(Uabc (pu))
  CFPREV/1(AMIN_CFPREV (deg)) -> AMIN_CFPREV (deg)/1

== system LF_AC29bus_HVDCdemo_V2_1/HVDC_network_avg/Inverter Control and Protection (Average model)/Inverter Protections/Informations ==
  note: The CFPREV  mitigates commutation failures due to AC voltage dips. After a fault detection (three-phase or
      | one-phase) an angle value (AMIN_CFPREV) is sent to the converter control in order to be deducted from the
      | maximum delay angle limit (alpha_max). In practice, the commutation margin is consequently enlarged
      | reducing therefore the risk of commutation failures (note 1).
  note: The Commutation failure prevention control (CFPREV) and the Low AC voltage detection (LACVD)
      | constitutes the protective functions at the rinverter.
  note: The LACVD detects a low AC voltage condition on the inverter commutation bus and sends a signal
      | (Lock) to the DCPROT (in the rectifier) in order to prevent the detection of a DC fault when the drop in
      | the DC voltage is due to a fault on the AC side. The LACVD at the irectifier sends also a signal to
      | lock the DCPROT for the same reason.
  note: DESCRIPTION
  note: DC Protections - Inverter
  note: NOTE 1: Result of a failure of the incoming valve to take over the direct current before the commutating voltage reverses its polarity.

== system LF_AC29bus_HVDCdemo_V2_1/HVDC_network_avg/Inverter Control and Protection (Average model)/Inverter Protections/Low  AC Voltage Detection (LACVD) ==
  note: Low AC Voltage Detection
  Uac (pu) : Inport
  Enable (Held) : EnablePort  PropagateVarSize=During execution  ShowOutputPort=on
  C : Constant  Value=STATE
  LACVD : Subsystem  TreatAsAtomicUnit=on
  Logical Operator : Logic  AllPortsSameDT=off
  Low_AC_Voltage : Outport
  wires:
  Uac (pu)/1 -> LACVD/1(Uac (pu))
  LACVD/1(Low_AC_Voltage) -> Low_AC_Voltage/1
  Enable (Held)/1 -> Logical Operator/1
  Logical Operator/1 -> LACVD/Enable
  C/1 -> Logical Operator/2

== system LF_AC29bus_HVDCdemo_V2_1/HVDC_network_avg/Inverter Control and Protection (Average model)/Inverter Protections/Udio_6p ==
  note: Three-phase full-wave rectification
  Uabc (pu) : Inport
  MinMax : MinMax  Function=max  SaturateOnIntegerOverflow=on  InputSameDT=on
  MinMax1 : MinMax  SaturateOnIntegerOverflow=on  InputSameDT=on
  Sum : Sum  Inputs=+-  SaturateOnIntegerOverflow=on  InputSameDT=on  OutDataTypeStr=Inherit: Same as first input
  conversion pu ac->dc : Gain  Gain=pi/(3*sqrt(3))  SaturateOnIntegerOverflow=on  OutDataTypeStr=Inherit: Same as input  ParamDataTypeStr=Inherit: Same as input
  Udio_6p : Outport
  wires:
  conversion pu ac->dc/1 -> Udio_6p/1
  Sum/1 -> conversion pu ac->dc/1
  Uabc (pu)/1 -> MinMax1/1, MinMax/1
  MinMax/1 -> Sum/1
  MinMax1/1 -> Sum/2

== system LF_AC29bus_HVDCdemo_V2_1/HVDC_network_avg/Master Control/Start//Stop/S1 ==
  Start : Inport
  Down : Constant  Value=0
  Ramp : FromWorkspace  VariableName="[T_ramp,  U_ramp]"  SampleTime=Ts
  Start-Stop Ramp : RateLimiter  RisingSlewLimit=SS_ramp  FallingSlewLimit=-SS_ramp
  Sum : Sum  SaturateOnIntegerOverflow=on  InputSameDT=on  OutDataTypeStr=Inherit: Same as first input
  Switch : Switch  Criteria=u2 > Threshold  SaturateOnIntegerOverflow=on
  UP : Constant  Value=Min_ref
  Out1 : Outport  InitialOutput=0
  wires:
  Sum/1 -> Out1/1
  Ramp/1 -> Sum/1
  Start/1 -> Switch/2
  Switch/1 -> Start-Stop Ramp/1
  Down/1 -> Switch/3
  UP/1 -> Switch/1
  Start-Stop Ramp/1 -> Sum/2

== system LF_AC29bus_HVDCdemo_V2_1/HVDC_network_avg/Rectifier Average model/HVDC_CONV_AVG/3-phase Current Source ==
  note: Ic = -(Ia + Ib)
  Iab : Inport
  Controlled Current Source : powerlib/Electrical Sources/Controlled Current Source  Initialize=off  Source_Type=AC  Amplitude=0  Phase=0  Frequency=0  Measurements=None
      settings: SourceProductName=Simscape Electrical
  Controlled Current Source1 : powerlib/Electrical Sources/Controlled Current Source  Initialize=off  Source_Type=AC  Amplitude=0  Phase=0  Frequency=0  Measurements=None
      settings: SourceProductName=Simscape Electrical
  Demux : Demux  Outputs=2
  A : PMIOPort  Side=Left
  B : PMIOPort  Port=2  Side=Left
  C : PMIOPort  Port=3  Side=Left
  wires:
  Iab/1 -> Demux/1
  Demux/1 -> Controlled Current Source/1
  Demux/2 -> Controlled Current Source1/1
  connections:
  A/RConn1 -- Controlled Current Source/LConn1
  B/RConn1 -- Controlled Current Source1/LConn1
  C/RConn1 -- Controlled Current Source1/RConn1 -- Controlled Current Source/RConn1

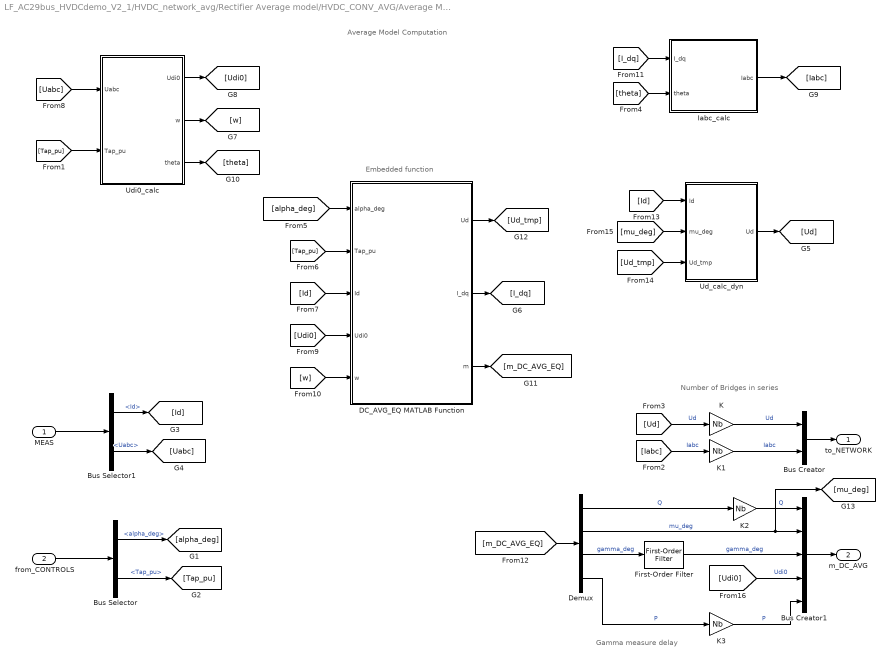
== system LF_AC29bus_HVDCdemo_V2_1/HVDC_network_avg/Rectifier Average model/HVDC_CONV_AVG/Average Model Computation ==
  note: Embedded function
  note: Gamma measure delay
  note: Average Model Computation
  note: Number of Bridges
      | in series
  MEAS : Inport
  from_CONTROLS : Inport  Port=2
  Bus Creator : BusCreator  Inputs=2
  Bus Creator1 : BusCreator  Inputs=5
  Bus Selector : BusSelector  OutputSignals=alpha_deg,Tap_pu
  Bus Selector1 : BusSelector  OutputSignals=Id,Uabc
  DC_AVG_EQ MATLAB Function : MATLAB Function  TreatAsAtomicUnit=on
  Demux : Demux
  First-Order Filter : powerlib_meascontrol/Filters/First-Order Filter  FilterType=Lowpass  Tc=1/(6*fn*2*pi)  Ts=Ts  Initialize=off  Vac_Init=[0, 0, 60]  Vdc_Init=0  PlotResponse=off  FreqRange="[0,  200,  1]"
      settings: SourceProductName=Simscape Electrical
  Iabc_calc : Subsystem
  K{,1..3} (4 alike) : Gain  Gain=Nb
  Ud_calc_dyn : Subsystem
  Udi0_calc : Subsystem
  to_NETWORK : Outport
  m_DC_AVG : Outport  Port=2
  wires:
  K3/1 -> Bus Creator1/5  "P"
  Demux/4 -> K3/1  "P"
  First-Order Filter/1 -> Bus Creator1/3  "gamma_deg"
  Demux/3 -> First-Order Filter/1  "gamma_deg"
  [Udi0] -> Bus Creator1/4  "Udi0"
  [mu_deg] -> Ud_calc_dyn/2(mu_deg)
  [Ud_tmp] -> Ud_calc_dyn/3(Ud_tmp)
  DC_AVG_EQ MATLAB Function/1(Ud) -> [Ud_tmp]
  Ud_calc_dyn/1(Ud) -> [Ud]
  [Id] -> Ud_calc_dyn/1(Id)
  K2/1 -> Bus Creator1/1  "Q"
  [w] -> DC_AVG_EQ MATLAB Function/5(w)
  [Udi0] -> DC_AVG_EQ MATLAB Function/4(Udi0)
  [Id] -> DC_AVG_EQ MATLAB Function/3(Id)
  [Uabc] -> Udi0_calc/1(Uabc)
  Bus Selector/1 -> [alpha_deg]  "<alpha_deg>"
  from_CONTROLS/1 -> Bus Selector/1
  Bus Selector/2 -> [Tap_pu]  "<Tap_pu>"
  MEAS/1 -> Bus Selector1/1
  Bus Selector1/1 -> [Id]  "<Id>"
  Bus Selector1/2 -> [Uabc]  "<Uabc>"
  [Tap_pu] -> Udi0_calc/2(Tap_pu)
  Bus Creator/1 -> to_NETWORK/1
  [Iabc] -> K1/1  "Iabc"
  [Ud] -> K/1  "Ud"
  K/1 -> Bus Creator/1  "Ud"
  K1/1 -> Bus Creator/2  "Iabc"
  Udi0_calc/2(w) -> [w]
  Udi0_calc/1(Udi0) -> [Udi0]
  Iabc_calc/1(Iabc) -> [Iabc]
  Udi0_calc/3(theta) -> [theta]
  [theta] -> Iabc_calc/2(theta)
  [I_dq] -> Iabc_calc/1(I_dq)
  [alpha_deg] -> DC_AVG_EQ MATLAB Function/1(alpha_deg)
  [Tap_pu] -> DC_AVG_EQ MATLAB Function/2(Tap_pu)
  DC_AVG_EQ MATLAB Function/2(I_dq) -> [I_dq]
  DC_AVG_EQ MATLAB Function/3(m) -> [m_DC_AVG_EQ]
  [m_DC_AVG_EQ] -> Demux/1
  Demux/1 -> K2/1  "Q"
  Demux/2 -> [mu_deg], Bus Creator1/2  "mu_deg"
  Bus Creator1/1 -> m_DC_AVG/1

== system LF_AC29bus_HVDCdemo_V2_1/HVDC_network_avg/Rectifier Average model/HVDC_CONV_AVG/CF_alarm ==
  note: CF_alarm
  note: Converter is deblocked
  Pd : Inport
  Udi0 : Inport  Port=2
  gamma_deg : Inport  Port=3
  Abs : Abs
  KPn : Constant  Value=Pn*Nb*0.05
  Logical Operator : Logic  Operator=OR  AllPortsSameDT=off  OutDataTypeStr=boolean
  Logical Operator1 : Logic  AllPortsSameDT=off  OutDataTypeStr=boolean
  Monostable : powerlib_meascontrol/Logic/Monostable  EdgeDetect=Rising  PulseDuration=T_alarm  ic=0  Ts=Ts
      settings: SourceProductName=Simscape Electrical  SourceProductBaseCode=PS
  Off Delay1 (T=1.2/(2*fn)) : powerlib_meascontrol/Logic/On Delay  DelayType=Off delay  delay=1.2/(2*fn)  ic=0  Ts=Ts
      settings: SourceProductName=Simscape Electrical
  Off Delay2 : powerlib_meascontrol/Logic/On Delay  DelayType=Off delay  delay=0.1  ic=0  Ts=Ts
      settings: SourceProductName=Simscape Electrical
  On Delay1 (T=2*Ts) : powerlib_meascontrol/Logic/On Delay  DelayType=On delay  delay=2*Ts  ic=0  Ts=Ts
      settings: SourceProductName=Simscape Electrical
  On Delay2 (T=1.5/(2*fn)) : powerlib_meascontrol/Logic/On Delay  DelayType=On delay  delay=1.5/(2*fn)  ic=0  Ts=Ts
      settings: SourceProductName=Simscape Electrical
  On Delay3 (T=1/fn) : powerlib_meascontrol/Logic/On Delay  DelayType=On delay  delay=1/fn  ic=0  Ts=Ts
      settings: SourceProductName=Simscape Electrical
  Relational Operator : RelationalOperator  Operator=<=  OutDataTypeStr=boolean  RndMeth=Nearest
  Relational Operator1 : RelationalOperator  Operator=<=  OutDataTypeStr=boolean  RndMeth=Nearest
  Relational Operator2 : RelationalOperator  OutDataTypeStr=boolean  RndMeth=Nearest
  Uac_min_lim : Constant  Value=0.8
  Udio_V->pu : Gain  Gain=1/((3*sqrt(2)/pi) * Usec)
  gamma_min_lim : Constant  Value=10
  CF_alarm : Outport
  wires:
  Off Delay2/1 -> Logical Operator1/2
  Abs/1 -> Relational Operator2/1
  Logical Operator1/1 -> Logical Operator/1
  On Delay2 (T=1.5/(2*fn))/1 -> Logical Operator1/1  "low_ac"
  Relational Operator2/1 -> Off Delay2/1
  KPn/1 -> Relational Operator2/2
  Pd/1 -> Abs/1
  On Delay3 (T=1/fn)/1 -> Logical Operator/2  "gamm_lim"
  Relational Operator1/1 -> On Delay3 (T=1/fn)/1
  gamma_min_lim/1 -> Relational Operator1/2
  gamma_deg/1 -> Relational Operator1/1
  Udio_V->pu/1 -> Relational Operator/1
  Uac_min_lim/1 -> Relational Operator/2
  Udi0/1 -> Udio_V->pu/1
  Relational Operator/1 -> On Delay1 (T=2*Ts)/1
  Off Delay1 (T=1.2/(2*fn))/1 -> On Delay2 (T=1.5/(2*fn))/1
  On Delay1 (T=2*Ts)/1 -> Off Delay1 (T=1.2/(2*fn))/1
  Logical Operator/1 -> Monostable/1
  Monostable/1 -> CF_alarm/1

== system LF_AC29bus_HVDCdemo_V2_1/HVDC_network_avg/Rectifier Control and Protection (Average model)/Rectifier Pole Control (Current)/Alpha Control ==
  note: Alpha Control
  Forced_alpha : Inport
  D_alpha : Inport  Port=2
  Constant1 : Constant  Value=alpha_min
  Constant2 : Constant  Value=alpha_max
  Constant3 : Constant  Value=test_alpha
  Data Type Conversion : DataTypeConversion  OutDataTypeStr=boolean  SaturateOnIntegerOverflow=on  RndMeth=Zero
  Logical Operator : Logic  Operator=OR
  "Rate Limiter (Rate limit) " : RateLimiter  RisingSlewLimit=PRate_fix  FallingSlewLimit=NRate_fix
  "Rate Limiter (Rate limit)    " : RateLimiter  RisingSlewLimit=PRate_fix  FallingSlewLimit=NRate_fix
  Sum : Sum  Inputs=-+  SaturateOnIntegerOverflow=on  InputSameDT=on  OutDataTypeStr=Inherit: Same as first input
  Switch : Switch  Criteria=u2 > Threshold  SaturateOnIntegerOverflow=on  InputSameDT=on
  Switch1 : Switch  Criteria=u2 > Threshold  SaturateOnIntegerOverflow=on  InputSameDT=on
  fixed alpha (deg) : Constant  Value=alpha_fix
  Max_i : Outport
  Min_i : Outport  Port=2
  wires:
  "Rate Limiter (Rate limit)    "/1 -> Min_i/1
  "Rate Limiter (Rate limit) "/1 -> Max_i/1
  D_alpha/1 -> Sum/1
  Sum/1 -> Switch/3
  Constant2/1 -> Sum/2
  Constant3/1 -> Logical Operator/1
  Logical Operator/1 -> Switch/2, Switch1/2
  Constant1/1 -> Switch1/3
  Switch/1 -> "Rate Limiter (Rate limit) "/1
  Switch1/1 -> "Rate Limiter (Rate limit)    "/1
  fixed alpha (deg)/1 -> Switch/1, Switch1/1
  Forced_alpha/1 -> Data Type Conversion/1
  Data Type Conversion/1 -> Logical Operator/2
